simulink model "psbwindgen"  (Simulink 6.0)
settings: Solver=ode23tb  StartTime=0.0  StopTime=3  RelTol=1e-4
PreLoadFcn:
  | load psbwindgen_data
InitFcn:
  | powericon('psbinitsys',bdroot);
values from neighbouring files (symbols this model uses):
  psbwindgen_char = [0 0 0 0 0 0 0 0 0 0 0.02551 0.02551 ... (243 elements, 9x27)]    [power_windgen_init.mat]
undefined symbols (not defined in the file or in its folder): gcbh, powericon
libraries: powerlib2 x50, powerlib_extras x5
(part 2 of 2)

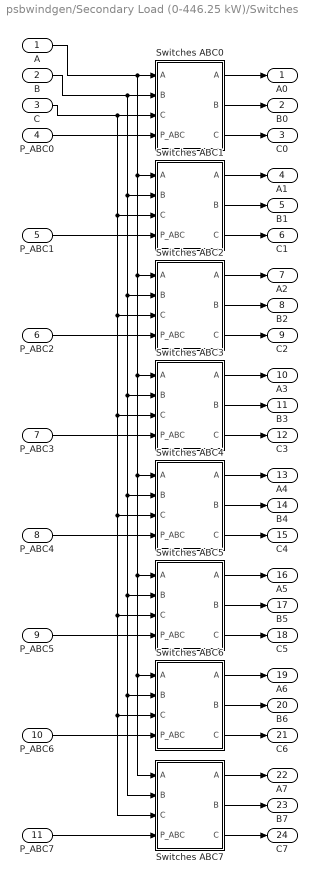
== system psbwindgen/Secondary Load (0-446.25 kW)/Switches ==
  A : Inport  Port=1  LatchInput=off
  B : Inport  Port=2  LatchInput=off
  C : Inport  Port=3  LatchInput=off
  P_ABC0 : Inport  Port=4  LatchInput=off
  P_ABC1 : Inport  Port=5  LatchInput=off
  P_ABC2 : Inport  Port=6  LatchInput=off
  P_ABC3 : Inport  Port=7  LatchInput=off
  P_ABC4 : Inport  Port=8  LatchInput=off
  P_ABC5 : Inport  Port=9  LatchInput=off
  P_ABC6 : Inport  Port=10  LatchInput=off
  P_ABC7 : Inport  Port=11  LatchInput=off
  Switches ABC0 : Subsystem
  Switches ABC1 : Subsystem
  Switches ABC2 : Subsystem
  Switches ABC3 : Subsystem
  Switches ABC4 : Subsystem
  Switches ABC5 : Subsystem
  Switches ABC6 : Subsystem
  Switches ABC7 : Subsystem
  A0 : Outport
  B0 : Outport  Port=2
  C0 : Outport  Port=3
  A1 : Outport  Port=4
  B1 : Outport  Port=5
  C1 : Outport  Port=6
  A2 : Outport  Port=7
  B2 : Outport  Port=8
  C2 : Outport  Port=9
  A3 : Outport  Port=10
  B3 : Outport  Port=11
  C3 : Outport  Port=12
  A4 : Outport  Port=13
  B4 : Outport  Port=14
  C4 : Outport  Port=15
  A5 : Outport  Port=16
  B5 : Outport  Port=17
  C5 : Outport  Port=18
  A6 : Outport  Port=19
  B6 : Outport  Port=20
  C6 : Outport  Port=21
  A7 : Outport  Port=22
  B7 : Outport  Port=23
  C7 : Outport  Port=24
  wires:
  P_ABC7/1 -> Switches ABC7/4(P_ABC)
  P_ABC6/1 -> Switches ABC6/4(P_ABC)
  P_ABC5/1 -> Switches ABC5/4(P_ABC)
  P_ABC4/1 -> Switches ABC4/4(P_ABC)
  P_ABC3/1 -> Switches ABC3/4(P_ABC)
  P_ABC2/1 -> Switches ABC2/4(P_ABC)
  P_ABC1/1 -> Switches ABC1/4(P_ABC)
  P_ABC0/1 -> Switches ABC0/4(P_ABC)
  C/1 -> Switches ABC6/3(C), Switches ABC7/3(C), Switches ABC5/3(C), Switches ABC4/3(C), Switches ABC3/3(C), Switches ABC2/3(C), Switches ABC1/3(C), Switches ABC0/3(C)
  B/1 -> Switches ABC6/2(B), Switches ABC7/2(B), Switches ABC5/2(B), Switches ABC4/2(B), Switches ABC3/2(B), Switches ABC2/2(B), Switches ABC1/2(B), Switches ABC0/2(B)
  A/1 -> Switches ABC6/1(A), Switches ABC7/1(A), Switches ABC5/1(A), Switches ABC4/1(A), Switches ABC3/1(A), Switches ABC2/1(A), Switches ABC1/1(A), Switches ABC0/1(A)
  Switches ABC7/3("C ") -> C7/1
  Switches ABC7/2("B ") -> B7/1
  Switches ABC7/1("A ") -> A7/1
  Switches ABC6/3("C ") -> C6/1
  Switches ABC6/2("B ") -> B6/1
  Switches ABC6/1("A ") -> A6/1
  Switches ABC5/3("C ") -> C5/1
  Switches ABC5/2("B ") -> B5/1
  Switches ABC5/1("A ") -> A5/1
  Switches ABC4/3("C ") -> C4/1
  Switches ABC4/2("B ") -> B4/1
  Switches ABC4/1("A ") -> A4/1
  Switches ABC3/3("C ") -> C3/1
  Switches ABC3/2("B ") -> B3/1
  Switches ABC3/1("A ") -> A3/1
  Switches ABC2/3("C ") -> C2/1
  Switches ABC2/2("B ") -> B2/1
  Switches ABC2/1("A ") -> A2/1
  Switches ABC1/3("C ") -> C1/1
  Switches ABC1/2("B ") -> B1/1
  Switches ABC1/1("A ") -> A1/1
  Switches ABC0/3("C ") -> C0/1
  Switches ABC0/2("B ") -> B0/1
  Switches ABC0/1("A ") -> A0/1

== system psbwindgen/WT/Ia ==
  Out1 : Outport
  wires:
  [tp575138] -> Out1/1

== system psbwindgen/WT/Ib ==
  Out1 : Outport
  wires:
  [tp575139] -> Out1/1

== system psbwindgen/WT/Ic ==
  Out1 : Outport
  wires:
  [tp575140] -> Out1/1

== system psbwindgen/WT/Vb ==
  Out1 : Outport
  wires:
  [tp575136] -> Out1/1

== system psbwindgen/WT/Vc ==
  Out1 : Outport
  wires:
  [tp575137] -> Out1/1

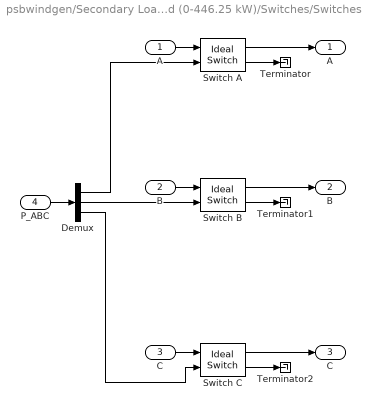
== system psbwindgen/Secondary Load (0-446.25 kW)/Switches/Switches ABC0 ==
  A : Inport  Port=1  LatchInput=off
  B : Inport  Port=2  LatchInput=off
  C : Inport  Port=3  LatchInput=off
  P_ABC : Inport  Port=4  LatchInput=off
  Demux : Demux  Outputs=3
  Switch A : powerlib2/Power Electronics/Ideal Switch  Tag=PoWeRsYsTeMbLoCk  Ron=Ron_switch  Lon=0  IC=Status(1)  Rs=Rs_snubber  Cs=Cs_snubber  PSBOutputType=10
  Switch B : powerlib2/Power Electronics/Ideal Switch  Tag=PoWeRsYsTeMbLoCk  Ron=Ron_switch  Lon=0  IC=Status(1)  Rs=Rs_snubber  Cs=Cs_snubber  PSBOutputType=10
  Switch C : powerlib2/Power Electronics/Ideal Switch  Tag=PoWeRsYsTeMbLoCk  Ron=Ron_switch  Lon=0  IC=Status(1)  Rs=Rs_snubber  Cs=Cs_snubber  PSBOutputType=10
  Terminator : Terminator
  Terminator1 : Terminator
  Terminator2 : Terminator
  "A " : Outport
  "B " : Outport  Port=2
  "C " : Outport  Port=3
  wires:
  Switch C/1 -> "C "/1
  Switch B/1 -> "B "/1
  Switch A/1 -> "A "/1
  C/1 -> Switch C/1
  B/1 -> Switch B/1
  P_ABC/1 -> Demux/1
  A/1 -> Switch A/1
  Demux/3 -> Switch C/2
  Demux/2 -> Switch B/2
  Demux/1 -> Switch A/2
  Switch C/2 -> Terminator2/1
  Switch B/2 -> Terminator1/1
  Switch A/2 -> Terminator/1

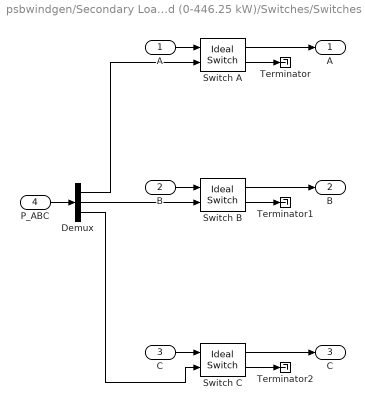
== system psbwindgen/Secondary Load (0-446.25 kW)/Switches/Switches ABC1 ==
  A : Inport  Port=1  LatchInput=off
  B : Inport  Port=2  LatchInput=off
  C : Inport  Port=3  LatchInput=off
  P_ABC : Inport  Port=4  LatchInput=off
  Demux : Demux  Outputs=3
  Switch A : powerlib2/Power Electronics/Ideal Switch  Tag=PoWeRsYsTeMbLoCk  Ron=Ron_switch  Lon=0  IC=Status(2)  Rs=Rs_snubber  Cs=Cs_snubber  PSBOutputType=10
  Switch B : powerlib2/Power Electronics/Ideal Switch  Tag=PoWeRsYsTeMbLoCk  Ron=Ron_switch  Lon=0  IC=Status(2)  Rs=Rs_snubber  Cs=Cs_snubber  PSBOutputType=10
  Switch C : powerlib2/Power Electronics/Ideal Switch  Tag=PoWeRsYsTeMbLoCk  Ron=Ron_switch  Lon=0  IC=Status(2)  Rs=Rs_snubber  Cs=Cs_snubber  PSBOutputType=10
  Terminator : Terminator
  Terminator1 : Terminator
  Terminator2 : Terminator
  "A " : Outport
  "B " : Outport  Port=2
  "C " : Outport  Port=3
  wires:
  Switch A/2 -> Terminator/1
  Switch B/2 -> Terminator1/1
  Switch C/2 -> Terminator2/1
  Demux/1 -> Switch A/2
  Demux/2 -> Switch B/2
  Demux/3 -> Switch C/2
  A/1 -> Switch A/1
  P_ABC/1 -> Demux/1
  B/1 -> Switch B/1
  C/1 -> Switch C/1
  Switch A/1 -> "A "/1
  Switch B/1 -> "B "/1
  Switch C/1 -> "C "/1

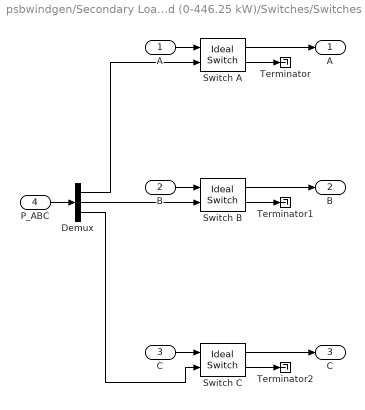
== system psbwindgen/Secondary Load (0-446.25 kW)/Switches/Switches ABC2 ==
  A : Inport  Port=1  LatchInput=off
  B : Inport  Port=2  LatchInput=off
  C : Inport  Port=3  LatchInput=off
  P_ABC : Inport  Port=4  LatchInput=off
  Demux : Demux  Outputs=3
  Switch A : powerlib2/Power Electronics/Ideal Switch  Tag=PoWeRsYsTeMbLoCk  Ron=Ron_switch  Lon=0  IC=Status(3)  Rs=Rs_snubber  Cs=Cs_snubber  PSBOutputType=10
  Switch B : powerlib2/Power Electronics/Ideal Switch  Tag=PoWeRsYsTeMbLoCk  Ron=Ron_switch  Lon=0  IC=Status(3)  Rs=Rs_snubber  Cs=Cs_snubber  PSBOutputType=10
  Switch C : powerlib2/Power Electronics/Ideal Switch  Tag=PoWeRsYsTeMbLoCk  Ron=Ron_switch  Lon=0  IC=Status(3)  Rs=Rs_snubber  Cs=Cs_snubber  PSBOutputType=10
  Terminator : Terminator
  Terminator1 : Terminator
  Terminator2 : Terminator
  "A " : Outport
  "B " : Outport  Port=2
  "C " : Outport  Port=3
  wires:
  Switch C/1 -> "C "/1
  Switch B/1 -> "B "/1
  Switch A/1 -> "A "/1
  C/1 -> Switch C/1
  B/1 -> Switch B/1
  P_ABC/1 -> Demux/1
  A/1 -> Switch A/1
  Demux/3 -> Switch C/2
  Demux/2 -> Switch B/2
  Demux/1 -> Switch A/2
  Switch C/2 -> Terminator2/1
  Switch B/2 -> Terminator1/1
  Switch A/2 -> Terminator/1

== system psbwindgen/Secondary Load (0-446.25 kW)/Switches/Switches ABC3 ==
  A : Inport  Port=1  LatchInput=off
  B : Inport  Port=2  LatchInput=off
  C : Inport  Port=3  LatchInput=off
  P_ABC : Inport  Port=4  LatchInput=off
  Demux : Demux  Outputs=3
  Switch A : powerlib2/Power Electronics/Ideal Switch  Tag=PoWeRsYsTeMbLoCk  Ron=Ron_switch  Lon=0  IC=Status(4)  Rs=Rs_snubber  Cs=Cs_snubber  PSBOutputType=10
  Switch B : powerlib2/Power Electronics/Ideal Switch  Tag=PoWeRsYsTeMbLoCk  Ron=Ron_switch  Lon=0  IC=Status(4)  Rs=Rs_snubber  Cs=Cs_snubber  PSBOutputType=10
  Switch C : powerlib2/Power Electronics/Ideal Switch  Tag=PoWeRsYsTeMbLoCk  Ron=Ron_switch  Lon=0  IC=Status(4)  Rs=Rs_snubber  Cs=Cs_snubber  PSBOutputType=10
  Terminator : Terminator
  Terminator1 : Terminator
  Terminator2 : Terminator
  "A " : Outport
  "B " : Outport  Port=2
  "C " : Outport  Port=3
  wires:
  Switch A/2 -> Terminator/1
  Switch B/2 -> Terminator1/1
  Switch C/2 -> Terminator2/1
  Demux/1 -> Switch A/2
  Demux/2 -> Switch B/2
  Demux/3 -> Switch C/2
  A/1 -> Switch A/1
  P_ABC/1 -> Demux/1
  B/1 -> Switch B/1
  C/1 -> Switch C/1
  Switch A/1 -> "A "/1
  Switch B/1 -> "B "/1
  Switch C/1 -> "C "/1

== system psbwindgen/Secondary Load (0-446.25 kW)/Switches/Switches ABC4 ==
  A : Inport  Port=1  LatchInput=off
  B : Inport  Port=2  LatchInput=off
  C : Inport  Port=3  LatchInput=off
  P_ABC : Inport  Port=4  LatchInput=off
  Demux : Demux  Outputs=3
  Switch A : powerlib2/Power Electronics/Ideal Switch  Tag=PoWeRsYsTeMbLoCk  Ron=Ron_switch  Lon=0  IC=Status(5)  Rs=Rs_snubber  Cs=Cs_snubber  PSBOutputType=10
  Switch B : powerlib2/Power Electronics/Ideal Switch  Tag=PoWeRsYsTeMbLoCk  Ron=Ron_switch  Lon=0  IC=Status(5)  Rs=Rs_snubber  Cs=Cs_snubber  PSBOutputType=10
  Switch C : powerlib2/Power Electronics/Ideal Switch  Tag=PoWeRsYsTeMbLoCk  Ron=Ron_switch  Lon=0  IC=Status(5)  Rs=Rs_snubber  Cs=Cs_snubber  PSBOutputType=10
  Terminator : Terminator
  Terminator1 : Terminator
  Terminator2 : Terminator
  "A " : Outport
  "B " : Outport  Port=2
  "C " : Outport  Port=3
  wires:
  Switch C/1 -> "C "/1
  Switch B/1 -> "B "/1
  Switch A/1 -> "A "/1
  C/1 -> Switch C/1
  B/1 -> Switch B/1
  P_ABC/1 -> Demux/1
  A/1 -> Switch A/1
  Demux/3 -> Switch C/2
  Demux/2 -> Switch B/2
  Demux/1 -> Switch A/2
  Switch C/2 -> Terminator2/1
  Switch B/2 -> Terminator1/1
  Switch A/2 -> Terminator/1

== system psbwindgen/Secondary Load (0-446.25 kW)/Switches/Switches ABC5 ==
  A : Inport  Port=1  LatchInput=off
  B : Inport  Port=2  LatchInput=off
  C : Inport  Port=3  LatchInput=off
  P_ABC : Inport  Port=4  LatchInput=off
  Demux : Demux  Outputs=3
  Switch A : powerlib2/Power Electronics/Ideal Switch  Tag=PoWeRsYsTeMbLoCk  Ron=Ron_switch  Lon=0  IC=Status(6)  Rs=Rs_snubber  Cs=Cs_snubber  PSBOutputType=10
  Switch B : powerlib2/Power Electronics/Ideal Switch  Tag=PoWeRsYsTeMbLoCk  Ron=Ron_switch  Lon=0  IC=Status(6)  Rs=Rs_snubber  Cs=Cs_snubber  PSBOutputType=10
  Switch C : powerlib2/Power Electronics/Ideal Switch  Tag=PoWeRsYsTeMbLoCk  Ron=Ron_switch  Lon=0  IC=Status(6)  Rs=Rs_snubber  Cs=Cs_snubber  PSBOutputType=10
  Terminator : Terminator
  Terminator1 : Terminator
  Terminator2 : Terminator
  "A " : Outport
  "B " : Outport  Port=2
  "C " : Outport  Port=3
  wires:
  Switch A/2 -> Terminator/1
  Switch B/2 -> Terminator1/1
  Switch C/2 -> Terminator2/1
  Demux/1 -> Switch A/2
  Demux/2 -> Switch B/2
  Demux/3 -> Switch C/2
  A/1 -> Switch A/1
  P_ABC/1 -> Demux/1
  B/1 -> Switch B/1
  C/1 -> Switch C/1
  Switch A/1 -> "A "/1
  Switch B/1 -> "B "/1
  Switch C/1 -> "C "/1

== system psbwindgen/Secondary Load (0-446.25 kW)/Switches/Switches ABC6 ==
  A : Inport  Port=1  LatchInput=off
  B : Inport  Port=2  LatchInput=off
  C : Inport  Port=3  LatchInput=off
  P_ABC : Inport  Port=4  LatchInput=off
  Demux : Demux  Outputs=3
  Switch A : powerlib2/Power Electronics/Ideal Switch  Tag=PoWeRsYsTeMbLoCk  Ron=Ron_switch  Lon=0  IC=Status(7)  Rs=Rs_snubber  Cs=Cs_snubber  PSBOutputType=10
  Switch B : powerlib2/Power Electronics/Ideal Switch  Tag=PoWeRsYsTeMbLoCk  Ron=Ron_switch  Lon=0  IC=Status(7)  Rs=Rs_snubber  Cs=Cs_snubber  PSBOutputType=10
  Switch C : powerlib2/Power Electronics/Ideal Switch  Tag=PoWeRsYsTeMbLoCk  Ron=Ron_switch  Lon=0  IC=Status(7)  Rs=Rs_snubber  Cs=Cs_snubber  PSBOutputType=10
  Terminator : Terminator
  Terminator1 : Terminator
  Terminator2 : Terminator
  "A " : Outport
  "B " : Outport  Port=2
  "C " : Outport  Port=3
  wires:
  Switch C/1 -> "C "/1
  Switch B/1 -> "B "/1
  Switch A/1 -> "A "/1
  C/1 -> Switch C/1
  B/1 -> Switch B/1
  P_ABC/1 -> Demux/1
  A/1 -> Switch A/1
  Demux/3 -> Switch C/2
  Demux/2 -> Switch B/2
  Demux/1 -> Switch A/2
  Switch C/2 -> Terminator2/1
  Switch B/2 -> Terminator1/1
  Switch A/2 -> Terminator/1

== system psbwindgen/Secondary Load (0-446.25 kW)/Switches/Switches ABC7 ==
  A : Inport  Port=1  LatchInput=off
  B : Inport  Port=2  LatchInput=off
  C : Inport  Port=3  LatchInput=off
  P_ABC : Inport  Port=4  LatchInput=off
  Demux : Demux  Outputs=3
  Switch A : powerlib2/Power Electronics/Ideal Switch  Tag=PoWeRsYsTeMbLoCk  Ron=Ron_switch  Lon=0  IC=Status(8)  Rs=Rs_snubber  Cs=Cs_snubber  PSBOutputType=10
  Switch B : powerlib2/Power Electronics/Ideal Switch  Tag=PoWeRsYsTeMbLoCk  Ron=Ron_switch  Lon=0  IC=Status(8)  Rs=Rs_snubber  Cs=Cs_snubber  PSBOutputType=10
  Switch C : powerlib2/Power Electronics/Ideal Switch  Tag=PoWeRsYsTeMbLoCk  Ron=Ron_switch  Lon=0  IC=Status(8)  Rs=Rs_snubber  Cs=Cs_snubber  PSBOutputType=10
  Terminator : Terminator
  Terminator1 : Terminator
  Terminator2 : Terminator
  "A " : Outport
  "B " : Outport  Port=2
  "C " : Outport  Port=3
  wires:
  Switch A/2 -> Terminator/1
  Switch B/2 -> Terminator1/1
  Switch C/2 -> Terminator2/1
  Demux/1 -> Switch A/2
  Demux/2 -> Switch B/2
  Demux/3 -> Switch C/2
  A/1 -> Switch A/1
  P_ABC/1 -> Demux/1
  B/1 -> Switch B/1
  C/1 -> Switch C/1
  Switch A/1 -> "A "/1
  Switch B/1 -> "B "/1
  Switch C/1 -> "C "/1
